simulink library "FFT"  (R2019a)
settings: Solver=VariableStepAuto  StartTime=0.0  StopTime=10.0  RelTol=1e-3
libraries: xbsIndex_r4 x2
settings Model: Creator=talon  LastModifiedBy=mybur

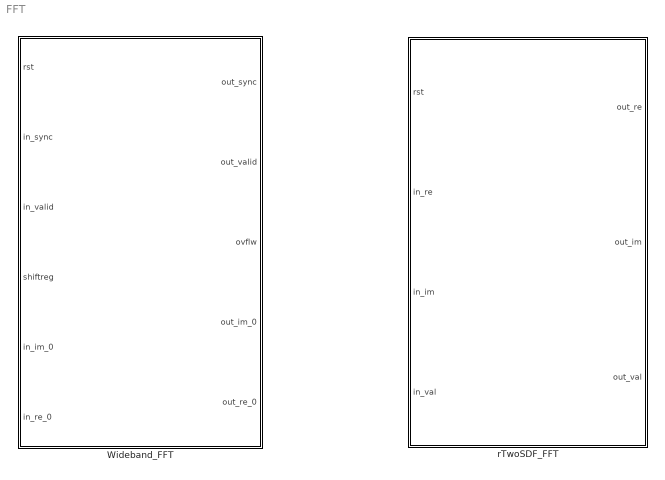
== system FFT ==
  Wideband_FFT : Subsystem  AncestorBlock=FFT/Wideband_FFT  mask{use_separate=on, use_fft_shift=off, use_reorder=on, wb_factor=1, twiddle_offset=0, nof_points=1024, xtra_dat_sigs=off, in_dat_w=9, out_dat_w=13, out_gain_w=0, stage_dat_w=18, guard_enable=off, guard_w=2, representation="SIGNED", use_round="ROUND", ovflw_behav="WRAP", use_dsp="YES", use_variant="4DSP", technology=0, ram_primitive="auto", fifo_primitive="auto"}
      mask prompts: use_separate "Separate complex in/out ports?"; use_fft_shift "Reorderder frequencies"; use_reorder "Bit reverse output"; wb_factor "Wideband factor"; twiddle_offset "Twiddle offsets"; nof_points "Number of points"; xtra_dat_sigs "Extra control signals"; in_dat_w "Input data width"; out_dat_w "Ouput data width"; out_gain_w "Output gain width"; stage_dat_w "Stage data width"; guard_enable "Guard enable"; guard_w "Guard bit width"; representation "Data Representation"; use_round "Rounding Behaviour"; ovflw_behav "Overflow Behaviour"; use_dsp "Use DSP for Cmults"; use_variant "Cmult options"; technology "Vendor (0-Xilinx, 1-Intel)"; ram_primitive "Ram Primitive"; fifo_primitive "Fifo Primitive"
      mask init:
      | Simulink.Block.eval([gcb, '/wb_fft']);
      | 
      | wb_fft_subsys2bb_knit();
      mask Callback use_separate:
      | enab = get_param(gcb,'use_separate');
      | 
      | % Set the 'MaskVisibilities' property for each parameters
      | if strcmp(enab,'on')
      |     set_param(gcb,'use_reorder','on');
      |     set_param(gcb,'use_fft_shift','off');
      |     set_param(gcb,'MaskEnables',{'on','off','off','on','on','on','on','on','on','on','on','on','on','on','on','on','on','on','on','on','on'});
      | else
      |     set_param(gcb,'MaskEnables',{'on','on','on','on','on','on','on','on','on','on','on','on','on','on','on','on','on','on','on','on','on'});
      | end
      mask Callback use_fft_shift:
      | enab = get_param(gcb,'use_fft_shift');
      | 
      | % Set the 'MaskVisibilities' property for each parameters
      | if strcmp(enab,'on')
      |     set_param(gcb,'use_reorder','on');
      |     set_param(gcb,'MaskEnables',{'on','on','off','on','on','on','on','on','on','on','on','on','on','on','on','on','on','on','on','on','on'});
      | else
      |     set_param(gcb,'MaskEnables',{'on','on','on','on','on','on','on','on','on','on','on','on','on','on','on','on','on','on','on','on','on'});
      | end
      mask Callback guard_enable:
      | enab = get_param(gcb,'guard_enable');
      | 
      | % Set the 'MaskVisibilities' property for each parameters
      | if strcmp(enab,'on')
      |     set_param(gcb,'MaskVisibilities',{'on','on','on','on','on','on','on','on','on','on','on','on','on','on','on','on','on','on','on','on','on'});
      | else
      |     set_param(gcb,'MaskVisibilities',{'on','on','on','on','on','on','on','on','on','on','on','on','off','on','on','on','on','on','on','on','on'});
      | end
      mask TypeOptions representation: "SIGNED" | "UNSIGNED"
      mask TypeOptions use_round: "ROUND" | "TRUNCTATE"
      mask TypeOptions ovflw_behav: "WRAP" | "SATURATE"
      mask TypeOptions use_dsp: "YES" | "NO"
      mask TypeOptions use_variant: "4DSP" | "3DSP"
      mask TypeOptions technology: 0 | 1
      mask TypeOptions ram_primitive: "auto" | "block" | "distributed" | "ultra"
      mask TypeOptions fifo_primitive: "auto" | "block" | "distributed" | "ultra"
      mask DialogControl fft_params Prompt: FFT Parameters
      mask DialogControl data_params Prompt: Data Parameters
      mask DialogControl synth_imp Prompt: FPGA Synth/Imp
  rTwoSDF_FFT : Subsystem  mask{g_nof_chan=0, g_use_reorder=on, g_in_dat_w=8, g_out_dat_w=14, g_stage_dat_w=18, g_guard_w=2, g_nof_points=512, g_variant="4DSP", g_use_dsp="yes", g_technology=0, g_ram_primitive="auto"}
      mask prompts: g_nof_chan "Number of channels"; g_use_reorder "Reorder output"; g_in_dat_w "Input data width"; g_out_dat_w "Output data width"; g_stage_dat_w "Stage data width"; g_guard_w "Guard bit width"; g_nof_points "Number of points"; g_variant "3 or 4 DSP for cmults"; g_use_dsp "Use DSP for cmults"; g_technology "Vendor (0-Xilinx, 1-Alterra)"; g_ram_primitive "Ram Primitive"
      mask TypeOptions g_variant: "3DSP" | "4DSP"
      mask TypeOptions g_use_dsp: "yes" | "no"
      mask TypeOptions g_technology: 0 | 1
      mask TypeOptions g_ram_primitive: "auto" | "distributed" | "block" | "ultra"

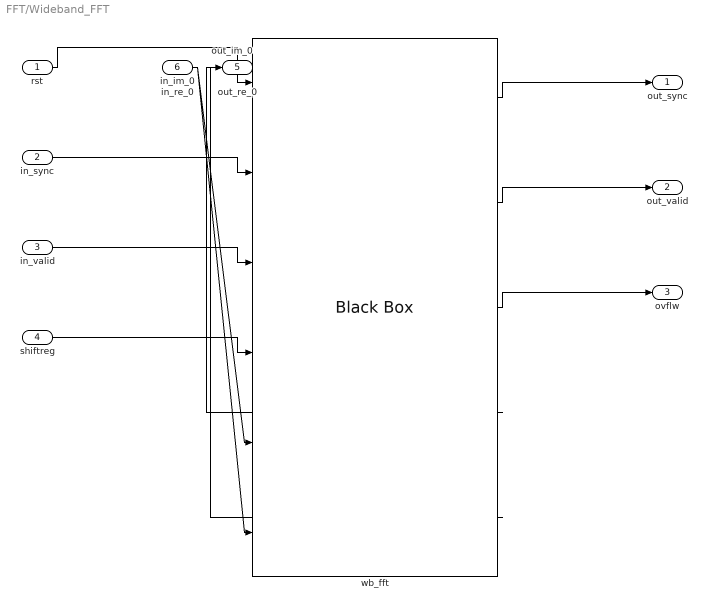
== system FFT/Wideband_FFT ==
  rst : Inport
  in_sync : Inport  Port=2
  in_valid : Inport  Port=3
  shiftreg : Inport  Port=4
  in_im_0 : Inport  Port=5
  in_re_0 : Inport  Port=6
  wb_fft : xbsIndex_r4/Black Box  init_code=casper_wb_fft_config  sim_method=ISE Simulator  verbose=off  block_type=blackbox2
  out_sync : Outport
  out_valid : Outport  Port=2
  ovflw : Outport  Port=3
  out_im_0 : Outport  Port=4
  out_re_0 : Outport  Port=5
  wires:
  wb_fft/5 -> out_re_0/1
  wb_fft/4 -> out_im_0/1
  in_re_0/1 -> wb_fft/6
  in_im_0/1 -> wb_fft/5
  wb_fft/3 -> ovflw/1
  shiftreg/1 -> wb_fft/4
  wb_fft/2 -> out_valid/1
  in_valid/1 -> wb_fft/3
  wb_fft/1 -> out_sync/1
  in_sync/1 -> wb_fft/2
  rst/1 -> wb_fft/1

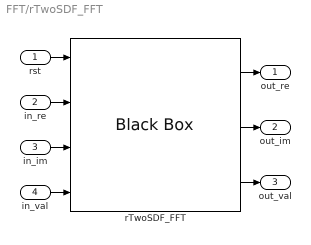
== system FFT/rTwoSDF_FFT ==
  rst : Inport
  in_re : Inport  Port=2
  in_im : Inport  Port=3
  in_val : Inport  Port=4
  rTwoSDF_FFT : xbsIndex_r4/Black Box  init_code=rTwoSDF_config  sim_method=ISE Simulator  verbose=off  block_type=blackbox2
  out_re : Outport
  out_im : Outport  Port=2
  out_val : Outport  Port=3
  wires:
  rTwoSDF_FFT/3 -> out_val/1
  in_im/1 -> rTwoSDF_FFT/3
  rst/1 -> rTwoSDF_FFT/1
  rTwoSDF_FFT/2 -> out_im/1
  in_re/1 -> rTwoSDF_FFT/2
  in_val/1 -> rTwoSDF_FFT/4
  rTwoSDF_FFT/1 -> out_re/1
